simulink model "assignment8"  (R2019a)
settings: Solver=VariableStepAuto  StartTime=0.0  StopTime=10.0  RelTol=1e-3
libraries: powerlib_meascontrol x1, simulink x1
settings Model: Creator=puja  LastModifiedBy=puja

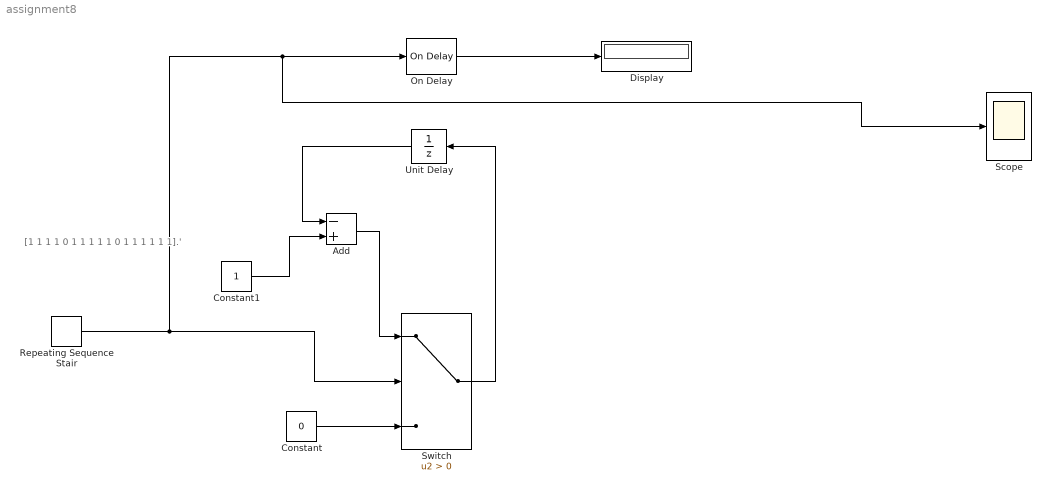
== system assignment8 ==
  note: [1 1 1 1 0 1 1 1 1 1 0 1 1 1 1 1 1].'
  Add : Sum  Inputs=-+
  Constant : Constant  Value=0
  Constant1 : Constant
  Display : Display
  On Delay : powerlib_meascontrol/Logic/On Delay  DelayType=On delay  delay=0.01  ic=0  Ts=0
      settings: SourceProductName=Simscape Electrical
  Repeating Sequence Stair : simulink/Sources/Repeating Sequence Stair  OutValues=[1 1 1 1 0 1 1 1 1 1 0 1 1 1 1 1 1].'  tsamp=-1  OutMin=[]  OutMax=[]  OutDataTypeStr=double  OutputDataTypeScalingMode=double  OutDataType=fixdt(0,8)  ConRadixGroup=Best Precision: Vector-wise  OutScaling=2^-12
  Scope : Scope
  Switch : Switch  Criteria=u2 > Threshold
  Unit Delay : UnitDelay  SampleTime=-1  HasFrameUpgradeWarning=on
  wires:
  Constant/1 -> Switch/3
  Add/1 -> Switch/1
  Constant1/1 -> Add/2
  Unit Delay/1 -> Add/1
  Switch/1 -> Unit Delay/1
  On Delay/1 -> Display/1
  Repeating Sequence Stair/1 -> Scope/1, On Delay/1, Switch/2
